simulink model "ROS_SL_Test_001"  (R2018b)
settings: Solver=VariableStepAuto  StartTime=0.0  StopTime=inf  FixedStep=0.1  RelTol=1e-3
libraries: robotlib x3
settings Model: Creator=USMAKRU  LastModifiedBy=USMAKRU

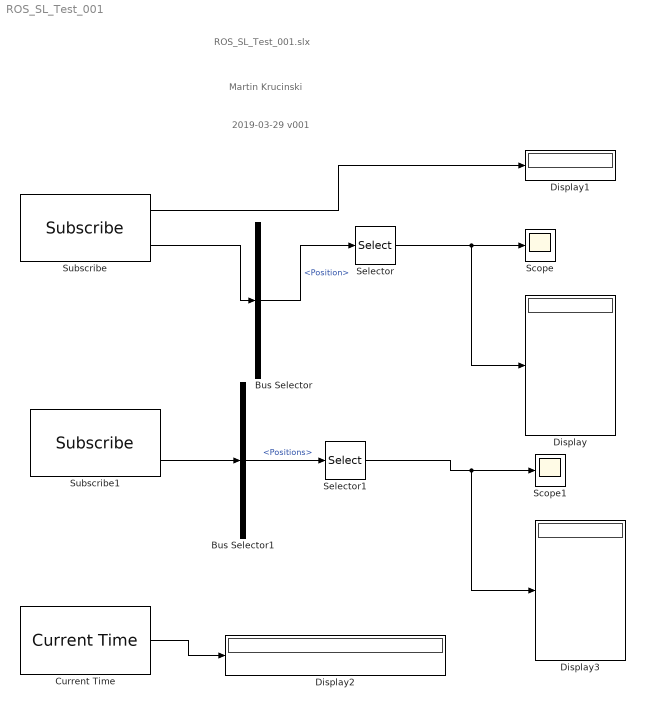
== system ROS_SL_Test_001 ==
  note: 2019-03-29 v001
  note: Martin Krucinski
  note: ROS_SL_Test_001.slx
  Bus Selector : BusSelector  OutputSignals=Position
  Bus Selector1 : BusSelector  OutputSignals=Actual.Positions
  Current Time : robotlib/Current Time  OutputFormat=double  SampleTime=-1  ModelName=ROS_SL_Test_001
      settings: SourceProductName=Robotics System Toolbox  SourceProductBaseCode=RO
  Display{,1..3} (4 alike) : Display
      Display2 settings: Format=hex (Stored Integer)
  Scope : Scope
  Scope1 : Scope
  Selector : Selector  InputPortWidth=128  IndexOptions=Index vector (dialog)  Indices=[1:6]  OutputSizes=1
  Selector1 : Selector  InputPortWidth=128  IndexOptions=Index vector (dialog)  Indices=[1:6]  OutputSizes=1
  Subscribe : robotlib/Subscribe  topicSource=Select from ROS network  topic=/joint_states  messageType=sensor_msgs/JointState  sampleTime=0.1  messageQueueLength=1
      settings: SourceProductBaseCode=RO
  Subscribe1 : robotlib/Subscribe  topicSource=Select from ROS network  topic=/feedback_states  messageType=control_msgs/FollowJointTrajectoryFeedback  sampleTime=0.1  messageQueueLength=1
      settings: SourceProductBaseCode=RO
  wires:
  Subscribe/2 -> Bus Selector/1
  Bus Selector/1 -> Selector/1  "<Position>"
  Subscribe/1 -> Display1/1
  Current Time/1 -> Display2/1
  Selector/1 -> Display/1, Scope/1
  Subscribe1/2 -> Bus Selector1/1
  Bus Selector1/1 -> Selector1/1  "<Positions>"
  Selector1/1 -> Display3/1, Scope1/1
